simulink model "multirotor_sim"  (R2021a)
settings: Solver=ode45  StartTime=0.0  StopTime=10  RelTol=1e-9  SampleTimeConstraint=STIndependent
values from neighbouring files (symbols this model uses):
  framePeriod_s = 1/frameRate_hz    (= 0.02)    [autocode_setup.m]    (also in setup.m)
undefined symbols (not defined in the file or in its folder): Aircraft, datetime, datevec, Earth, Env, Fmu, InitCond, Telem, WGS84
libraries: simulink x8, aerolibconvert2 x5, simulink_extras x4, aerolibtransform2 x3, aerolibasang x3, aerolibgravity2 x2, sharedtransform x1, aerolibatmos2 x1, uavutilslib x1, shared6dof x1
(part 2 of 3)

== system multirotor_sim/Flight Management Unit/Control Laws/Variant Subsystem/FMU v2 ==
  System Data : Inport
  Sensor Data : Inport  Port=2
  Navigation Filter Data : Inport  Port=3
  Telemetry Data : Inport  Port=4
  Flight Code : ModelReference  ModelNameDialog=fmu_v2.slx  SimulationMode=Normal  ModelReferenceVersion=2.2
  Virtual to Non-Virtual Mapping : Subsystem
  Virtual to Non-Virtual Mapping1 : Subsystem
  Virtual to Non-Virtual Mapping2 : Subsystem
  Virtual to Non-Virtual Mapping3 : Subsystem
  Virtual to Non-Virtual Mapping4 : Subsystem
  Control Data : Outport
  wires:
  Virtual to Non-Virtual Mapping3/1(Non-Virtual) -> Flight Code/4
  Sensor Data/1 -> Virtual to Non-Virtual Mapping1/1(Virtual)
  Virtual to Non-Virtual Mapping4/1(Virtual) -> Control Data/1
  Virtual to Non-Virtual Mapping/1(Non-Virtual) -> Flight Code/1
  Flight Code/1 -> Virtual to Non-Virtual Mapping4/1(Non-Virtual)
  System Data/1 -> Virtual to Non-Virtual Mapping/1(Virtual)
  Navigation Filter Data/1 -> Virtual to Non-Virtual Mapping2/1(Virtual)
  Virtual to Non-Virtual Mapping1/1(Non-Virtual) -> Flight Code/2
  Virtual to Non-Virtual Mapping2/1(Non-Virtual) -> Flight Code/3
  Telemetry Data/1 -> Virtual to Non-Virtual Mapping3/1(Virtual)

== system multirotor_sim/Flight Management Unit/Control Laws/Variant Subsystem/FMU v2 Beta ==
  System Data : Inport
  Sensor Data : Inport  Port=2
  Navigation Filter Data : Inport  Port=3
  Telemetry Data : Inport  Port=4
  Flight Code : ModelReference  ModelNameDialog=fmu_v2_beta.slx  SimulationMode=Normal  ModelReferenceVersion=2.1
  Virtual to Non-Virtual Mapping : Subsystem
  Virtual to Non-Virtual Mapping1 : Subsystem
  Virtual to Non-Virtual Mapping2 : Subsystem
  Virtual to Non-Virtual Mapping3 : Subsystem
  Virtual to Non-Virtual Mapping4 : Subsystem
  Control Data : Outport
  wires:
  Virtual to Non-Virtual Mapping3/1(Non-Virtual) -> Flight Code/4
  Sensor Data/1 -> Virtual to Non-Virtual Mapping1/1(Virtual)
  Virtual to Non-Virtual Mapping4/1(Virtual) -> Control Data/1
  Virtual to Non-Virtual Mapping/1(Non-Virtual) -> Flight Code/1
  Flight Code/1 -> Virtual to Non-Virtual Mapping4/1(Non-Virtual)
  System Data/1 -> Virtual to Non-Virtual Mapping/1(Virtual)
  Navigation Filter Data/1 -> Virtual to Non-Virtual Mapping2/1(Virtual)
  Virtual to Non-Virtual Mapping1/1(Non-Virtual) -> Flight Code/2
  Virtual to Non-Virtual Mapping2/1(Non-Virtual) -> Flight Code/3
  Telemetry Data/1 -> Virtual to Non-Virtual Mapping3/1(Virtual)

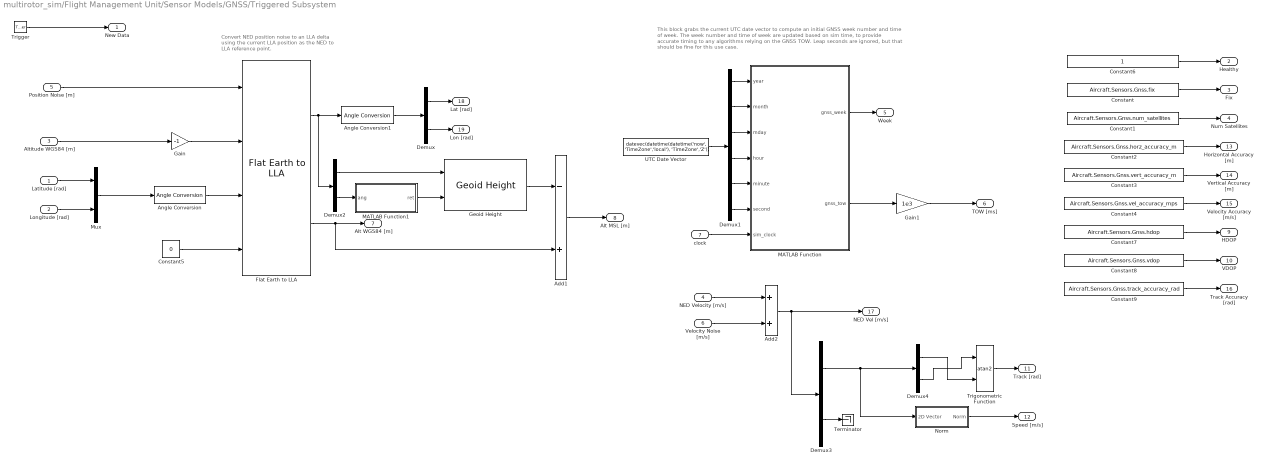
== system multirotor_sim/Flight Management Unit/Sensor Models/GNSS/Triggered Subsystem ==
  note: This block grabs the current UTC date vector to compute an initial GNSS week number
      | and time of week. The week number and time of week are updated based on sim time, to provide accurate timing to any algorithms relying on the GNSS TOW. Leap seconds are ignored, but that should be fine for this use case.
  note: Convert NED position noise to an LLA delta
      | using the current LLA position as the NED to
      | LLA reference point.
  Latitude [rad] : Inport
  "Longitude [rad] " : Inport  Port=2
  Altitude WGS84 [m] : Inport  Port=3
  NED Velocity [m/s] : Inport  Port=4  PortDimensions=3
  Position Noise [m] : Inport  Port=5  PortDimensions=3
  Velocity Noise [m/s] : Inport  Port=6  PortDimensions=3
  clock : Inport  Port=7
  Trigger : TriggerPort  VariantControl=Variant  ShowOutputPort=on
  Add1 : Sum  Inputs=-+
  Add2 : Sum
  Angle Conversion : aerolibconvert2/Angle Conversion  IU=rad  OU=deg
  Angle Conversion1 : aerolibconvert2/Angle Conversion  IU=deg  OU=rad
  Constant : Constant  Value=Aircraft.Sensors.Gnss.fix
  Constant1 : Constant  Value=Aircraft.Sensors.Gnss.num_satellites
  Constant2 : Constant  Value=Aircraft.Sensors.Gnss.horz_accuracy_m
  Constant3 : Constant  Value=Aircraft.Sensors.Gnss.vert_accuracy_m
  Constant4 : Constant  Value=Aircraft.Sensors.Gnss.vel_accuracy_mps
  Constant5 : Constant  Value=0
  Constant6 : Constant
  Constant7 : Constant  Value=Aircraft.Sensors.Gnss.hdop
  Constant8 : Constant  Value=Aircraft.Sensors.Gnss.vdop
  Constant9 : Constant  Value=Aircraft.Sensors.Gnss.track_accuracy_rad
  Demux : Demux  Outputs=2
  Demux1 : Demux  Outputs=6
  Demux2 : Demux  Outputs=2
  Demux3 : Demux  Outputs=[2 1]
  Demux4 : Demux  Outputs=2
  Flat Earth to LLA : aerolibtransform2/Flat Earth to LLA  units=Metric (MKS)  ptype=Earth (WGS84)  F=1/298.257223563  R=6378137  refPosPort=on  LL0=[0 10]  psi=0
  Gain : Gain  Gain=-1
  Gain1 : Gain  Gain=1e3
  Geoid Height : aerolibgravity2/Geoid Height  units=Metric (MKS)  gtype=EGM96  datafile='geoidegm96grid'  dtype=double  action=Warning
      settings: SourceProductBaseCode=AE
  MATLAB Function : MATLAB Function  TreatAsAtomicUnit=on
  MATLAB Function1 : MATLAB Function  TreatAsAtomicUnit=on
  Mux : Mux  Inputs=2
  Norm : Subsystem
  Terminator : Terminator
  Trigonometric Function : Trigonometry  Operator=atan2
  UTC Date Vector : Constant  Value=datevec(datetime(datetime('now', 'TimeZone','local'), 'TimeZone','Z'))  SampleTime=-1
  New Data : Outport
  Healthy : Outport  Port=2
  Fix : Outport  Port=3
  Num Satellites : Outport  Port=4
  Week : Outport  Port=5
  TOW [ms] : Outport  Port=6
  Alt WGS84 [m] : Outport  Port=7
  Alt MSL [m] : Outport  Port=8
  HDOP : Outport  Port=9
  VDOP : Outport  Port=10
  Track [rad] : Outport  Port=11
  Speed [m/s] : Outport  Port=12
  Horizontal Accuracy [m] : Outport  Port=13
  Vertical Accuracy [m] : Outport  Port=14
  Velocity Accuracy [m/s] : Outport  Port=15
  Track Accuracy [rad] : Outport  Port=16
  NED Vel [m/s] : Outport  Port=17
  Lat [rad] : Outport  Port=18
  Lon [rad] : Outport  Port=19
  wires:
  Constant/1 -> Fix/1
  Constant1/1 -> Num Satellites/1
  Constant2/1 -> Horizontal Accuracy [m]/1
  Constant3/1 -> Vertical Accuracy [m]/1
  Constant4/1 -> Velocity Accuracy [m/s]/1
  Position Noise [m]/1 -> Flat Earth to LLA/1
  Altitude WGS84 [m]/1 -> Gain/1
  Mux/1 -> Angle Conversion/1
  Angle Conversion/1 -> Flat Earth to LLA/3
  Constant5/1 -> Flat Earth to LLA/4
  "Longitude [rad] "/1 -> Mux/2
  Latitude [rad]/1 -> Mux/1
  Flat Earth to LLA/1 -> Demux2/1, Angle Conversion1/1
  Angle Conversion1/1 -> Demux/1
  Demux/2 -> Lon [rad]/1
  Demux/1 -> Lat [rad]/1
  Flat Earth to LLA/2 -> Add1/2, Alt WGS84 [m]/1
  NED Velocity [m/s]/1 -> Add2/1
  Add2/1 -> Demux3/1, NED Vel [m/s]/1
  Demux1/2 -> MATLAB Function/2(month)
  Demux1/6 -> MATLAB Function/6(second)
  UTC Date Vector/1 -> Demux1/1
  Demux1/1 -> MATLAB Function/1(year)
  Demux1/5 -> MATLAB Function/5(minute)
  Demux1/4 -> MATLAB Function/4(hour)
  Demux1/3 -> MATLAB Function/3(mday)
  MATLAB Function/2(gnss_tow) -> Gain1/1
  MATLAB Function/1(gnss_week) -> Week/1
  clock/1 -> MATLAB Function/7(sim_clock)
  Gain/1 -> Flat Earth to LLA/2
  Constant6/1 -> Healthy/1
  Trigger/1 -> New Data/1
  Gain1/1 -> TOW [ms]/1
  Demux2/1 -> Geoid Height/1
  Demux2/2 -> MATLAB Function1/1(ang)
  MATLAB Function1/1(ret) -> Geoid Height/2
  Geoid Height/1 -> Add1/1
  Add1/1 -> Alt MSL [m]/1
  Constant7/1 -> HDOP/1
  Constant8/1 -> VDOP/1
  Demux4/1 -> Trigonometric Function/2
  Demux4/2 -> Trigonometric Function/1
  Trigonometric Function/1 -> Track [rad]/1
  Velocity Noise [m/s]/1 -> Add2/2
  Constant9/1 -> Track Accuracy [rad]/1
  Demux3/1 -> Norm/1(2D Vector), Demux4/1
  Demux3/2 -> Terminator/1
  Norm/1(Norm) -> Speed [m/s]/1

== system multirotor_sim/Flight Management Unit/Sensor Models/IMU/Accelerometer ==
  Body Accel [m/s/s] : Inport  PortDimensions=3
  Gravitational Accel in Body Frame [m/s/s] : Inport  Port=2  PortDimensions=3
  Add : Sum  Inputs=+++
  Band-Limited White Noise : simulink/Sources/Band-Limited White Noise  Cov=Aircraft.Sensors.Imu.Accel.noise_mps2  Ts=0.1  seed=[23341]
  Constant : Constant  Value=Aircraft.Sensors.Imu.Accel.bias_mps2  VectorParams1D=off
  Constant1 : Constant  Value=Aircraft.Sensors.Imu.Accel.scale_factor
  Product : Product  Multiplication=Matrix(*)
  Reshape : Reshape  OutputDimensionality=Column vector (2-D)
  Reshape1 : Reshape  OutputDimensionality=Column vector (2-D)
  Reshape2 : Reshape
  Saturation : Saturate  UpperLimit=Aircraft.Sensors.Imu.Accel.upper_limit_mps2  LowerLimit=Aircraft.Sensors.Imu.Accel.lower_limit_mps2
  Subtract : Sum  Inputs=+-
  Accelerometer [m/s/s] : Outport  PortDimensions=3
  wires:
  Add/1 -> Saturation/1
  Band-Limited White Noise/1 -> Add/1
  Product/1 -> Add/3
  Constant/1 -> Add/2
  Constant1/1 -> Product/1
  Subtract/1 -> Product/2
  Reshape/1 -> Subtract/2
  Gravitational Accel in Body Frame [m/s/s]/1 -> Reshape/1
  Reshape1/1 -> Subtract/1
  Body Accel [m/s/s]/1 -> Reshape1/1
  Saturation/1 -> Reshape2/1
  Reshape2/1 -> Accelerometer [m/s/s]/1

== system multirotor_sim/Flight Management Unit/Sensor Models/IMU/Gyro ==
  Body Rotational Rate [rad/s] : Inport  PortDimensions=3
  Body Accel [m/s/s] : Inport  Port=2  PortDimensions=3
  Add1 : Sum  Inputs=++++
  Band-Limited White Noise : simulink/Sources/Band-Limited White Noise  Cov=Aircraft.Sensors.Imu.Gyro.noise_radps  Ts=0.1  seed=[23341]  VectorParams1D=off
  Constant1 : Constant  Value=Aircraft.Sensors.Imu.Gyro.bias_radps  VectorParams1D=off
  Constant2 : Constant  Value=Aircraft.Sensors.Imu.Gyro.accel_sens_radps
  Constant3 : Constant  Value=Aircraft.Sensors.Imu.Gyro.scale_factor  VectorParams1D=off
  Product : Product
  Product1 : Product  Multiplication=Matrix(*)
  Reshape : Reshape  OutputDimensionality=Column vector (2-D)
  Reshape1 : Reshape  OutputDimensionality=Column vector (2-D)
  Reshape2 : Reshape
  Saturation : Saturate  UpperLimit=Aircraft.Sensors.Imu.Gyro.upper_limit_radps  LowerLimit=Aircraft.Sensors.Imu.Gyro.lower_limit_radps
  Gyro [rad/s] : Outport  PortDimensions=3
  wires:
  Constant3/1 -> Product1/1
  Constant2/1 -> Product/1
  Add1/1 -> Saturation/1
  Constant1/1 -> Add1/3
  Product1/1 -> Add1/4
  Band-Limited White Noise/1 -> Add1/2
  Body Rotational Rate [rad/s]/1 -> Reshape/1
  Reshape/1 -> Product1/2
  Body Accel [m/s/s]/1 -> Product/2
  Product/1 -> Reshape1/1
  Reshape1/1 -> Add1/1
  Reshape2/1 -> Gyro [rad/s]/1
  Saturation/1 -> Reshape2/1

== system multirotor_sim/Flight Management Unit/Sensor Models/IMU/Magnetometer ==
  Body Magnetic Field [uT] : Inport  PortDimensions=3
  Add2 : Sum  Inputs=+++
  Band-Limited White Noise : simulink/Sources/Band-Limited White Noise  Cov=Aircraft.Sensors.Imu.Mag.noise_ut  Ts=0.1  seed=[23341]
  Constant1 : Constant  Value=Aircraft.Sensors.Imu.Mag.scale_factor  VectorParams1D=off
  Constant2 : Constant  Value=Aircraft.Sensors.Imu.Mag.bias_ut
  Product : Product  Multiplication=Matrix(*)
  Reshape : Reshape  OutputDimensionality=Column vector (2-D)
  Reshape1 : Reshape
  Saturation : Saturate  UpperLimit=Aircraft.Sensors.Imu.Mag.upper_limit_ut  LowerLimit=Aircraft.Sensors.Imu.Mag.lower_limit_ut
  Magnetometer [uT] : Outport  PortDimensions=3
  wires:
  Body Magnetic Field [uT]/1 -> Reshape/1
  Band-Limited White Noise/1 -> Add2/1
  Add2/1 -> Saturation/1
  Constant2/1 -> Add2/2
  Constant1/1 -> Product/1
  Reshape/1 -> Product/2
  Saturation/1 -> Reshape1/1
  Reshape1/1 -> Magnetometer [uT]/1
  Product/1 -> Add2/3

== system multirotor_sim/Vehicle/Forces and Moments/Propulsive/Mz calculation1 ==
  Motor_torque : Inport
  Constant : Constant  Value=Aircraft.Motor.dir
  MatrixMultiply : Product  Multiplication=Matrix(*)
  Mz_from_motor_torque : Outport
  wires:
  Motor_torque/1 -> MatrixMultiply/1
  Constant/1 -> MatrixMultiply/2
  MatrixMultiply/1 -> Mz_from_motor_torque/1

== system multirotor_sim/Flight Management Unit/Control Laws/Variant Subsystem/FMU v1/Virtual to Non-Virtual Mapping ==
  Virtual : Inport
  Bus Creator : BusCreator  Inputs=8  OutDataTypeStr=Bus: SysData  NonVirtualBus=on
  Bus Selector : BusSelector  OutputSignals=Frame Time [us],Frame Time [s],Input Voltage,Regulated Voltage,PWM Voltage,SBUS Voltage,System Time [us],System Time [s]
  Data Type Conversion : DataTypeConversion  OutDataTypeStr=int32
  Data Type Conversion{1..4,6} (5 alike) : DataTypeConversion  OutDataTypeStr=single
  Data Type Conversion5 : DataTypeConversion  OutDataTypeStr=int64
  Data Type Conversion7 : DataTypeConversion  OutDataTypeStr=double
  Non-Virtual : Outport  OutDataTypeStr=Bus: SysData
  wires:
  Data Type Conversion7/1 -> Bus Creator/8  "sys_time_s"
  Bus Selector/8 -> Data Type Conversion7/1  "<System Time [s]>"
  Data Type Conversion6/1 -> Bus Creator/2  "frame_time_s"
  Bus Selector/2 -> Data Type Conversion6/1  "<Frame Time [s]>"
  Data Type Conversion5/1 -> Bus Creator/7  "sys_time_us"
  Bus Selector/7 -> Data Type Conversion5/1  "<System Time [us]>"
  Data Type Conversion4/1 -> Bus Creator/6  "sbus_volt"
  Data Type Conversion3/1 -> Bus Creator/5  "pwm_volt"
  Data Type Conversion2/1 -> Bus Creator/4  "reg_volt"
  Bus Selector/6 -> Data Type Conversion4/1  "<SBUS Voltage>"
  Bus Selector/5 -> Data Type Conversion3/1  "<PWM Voltage>"
  Bus Selector/4 -> Data Type Conversion2/1  "<Regulated Voltage>"
  Data Type Conversion1/1 -> Bus Creator/3  "input_volt"
  Bus Selector/3 -> Data Type Conversion1/1  "<Input Voltage>"
  Data Type Conversion/1 -> Bus Creator/1  "frame_time_us"
  Bus Selector/1 -> Data Type Conversion/1  "<Frame Time [us]>"
  Virtual/1 -> Bus Selector/1
  Bus Creator/1 -> Non-Virtual/1

== system multirotor_sim/Flight Management Unit/Control Laws/Variant Subsystem/FMU v1/Virtual to Non-Virtual Mapping1 ==
  Virtual : Inport
  Bus Creator : BusCreator  Inputs=7  OutDataTypeStr=Bus: SensorData  NonVirtualBus=on
  Bus Selector : BusSelector  OutputSignals=Pitot Static Installed,Inceptor,IMU,GNSS,Static Pressure,Differential Pressure,Analog
  Data Type Conversion : DataTypeConversion  OutDataTypeStr=boolean
  Virtual to Non-Virtual Mapping1 : Subsystem
  Virtual to Non-Virtual Mapping2 : Subsystem
  Virtual to Non-Virtual Mapping3 : Subsystem
  Virtual to Non-Virtual Mapping4 : Subsystem
  Virtual to Non-Virtual Mapping5 : Subsystem
  Virtual to Non-Virtual Mapping6 : Subsystem
  Non-Virtual : Outport  OutDataTypeStr=Bus: SensorData
  wires:
  Virtual to Non-Virtual Mapping6/1(Non-Virtual) -> Bus Creator/7  "analog"
  Bus Selector/7 -> Virtual to Non-Virtual Mapping6/1(Virtual)  "<Analog>"
  Bus Selector/6 -> Virtual to Non-Virtual Mapping5/1(Virtual)  "<Differential Pressure>"
  Virtual to Non-Virtual Mapping5/1(Non-Virtual) -> Bus Creator/6  "diff_pres"
  Bus Selector/5 -> Virtual to Non-Virtual Mapping4/1(Virtual)  "<Static Pressure>"
  Virtual to Non-Virtual Mapping4/1(Non-Virtual) -> Bus Creator/5  "static_pres"
  Bus Selector/4 -> Virtual to Non-Virtual Mapping3/1(Virtual)  "<GNSS>"
  Virtual to Non-Virtual Mapping3/1(Non-Virtual) -> Bus Creator/4  "gnss"
  Bus Selector/3 -> Virtual to Non-Virtual Mapping2/1(Virtual)  "<IMU>"
  Virtual to Non-Virtual Mapping2/1(Non-Virtual) -> Bus Creator/3  "imu"
  Virtual to Non-Virtual Mapping1/1(Non-Virtual) -> Bus Creator/2  "inceptor"
  Bus Selector/2 -> Virtual to Non-Virtual Mapping1/1(Virtual)  "<Inceptor>"
  Data Type Conversion/1 -> Bus Creator/1  "pitot_static_installed"
  Bus Selector/1 -> Data Type Conversion/1  "<Pitot Static Installed>"
  Bus Creator/1 -> Non-Virtual/1
  Virtual/1 -> Bus Selector/1

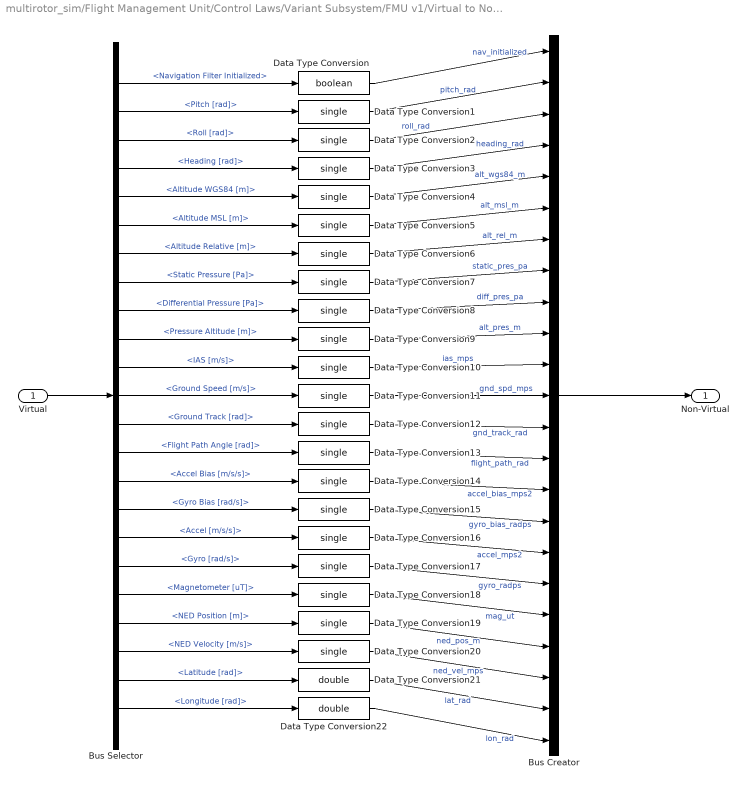
== system multirotor_sim/Flight Management Unit/Control Laws/Variant Subsystem/FMU v1/Virtual to Non-Virtual Mapping2 ==
  Virtual : Inport
  Bus Creator : BusCreator  Inputs=23  OutDataTypeStr=Bus: NavData  NonVirtualBus=on
  Bus Selector : BusSelector  OutputSignals=Navigation Filter Initialized,Pitch [rad],Roll [rad],Heading [rad],Altitude WGS84 [m],Altitude MSL [m],Altitude Relative [m],Static Pressure [Pa],Differential Pressure [Pa],Pressure Altitude [m],IAS [m/s],Ground Speed [m/s],Ground Track [rad],Flight Path Angle [rad],Accel Bias [m/s/s],Gyro Bias [rad/s],Accel [m/s/s],Gyro [rad/s],Magnetometer [uT],NED Position [m],NED Velocity [m/s],Latitude [rad],Longitude [rad]
  Data Type Conversion : DataTypeConversion  OutDataTypeStr=boolean
  Data Type Conversion{1..20} (20 alike) : DataTypeConversion  OutDataTypeStr=single
  Data Type Conversion21 : DataTypeConversion  OutDataTypeStr=double
  Data Type Conversion22 : DataTypeConversion  OutDataTypeStr=double
  Non-Virtual : Outport  OutDataTypeStr=Bus: NavData
  wires:
  Data Type Conversion17/1 -> Bus Creator/18  "gyro_radps"
  Data Type Conversion22/1 -> Bus Creator/23  "lon_rad"
  Data Type Conversion21/1 -> Bus Creator/22  "lat_rad"
  Data Type Conversion20/1 -> Bus Creator/21  "ned_vel_mps"
  Data Type Conversion19/1 -> Bus Creator/20  "ned_pos_m"
  Data Type Conversion18/1 -> Bus Creator/19  "mag_ut"
  Data Type Conversion16/1 -> Bus Creator/17  "accel_mps2"
  Data Type Conversion15/1 -> Bus Creator/16  "gyro_bias_radps"
  Data Type Conversion14/1 -> Bus Creator/15  "accel_bias_mps2"
  Data Type Conversion13/1 -> Bus Creator/14  "flight_path_rad"
  Data Type Conversion12/1 -> Bus Creator/13  "gnd_track_rad"
  Data Type Conversion11/1 -> Bus Creator/12  "gnd_spd_mps"
  Data Type Conversion10/1 -> Bus Creator/11  "ias_mps"
  Data Type Conversion9/1 -> Bus Creator/10  "alt_pres_m"
  Data Type Conversion8/1 -> Bus Creator/9  "diff_pres_pa"
  Data Type Conversion7/1 -> Bus Creator/8  "static_pres_pa"
  Data Type Conversion6/1 -> Bus Creator/7  "alt_rel_m"
  Data Type Conversion5/1 -> Bus Creator/6  "alt_msl_m"
  Data Type Conversion4/1 -> Bus Creator/5  "alt_wgs84_m"
  Data Type Conversion3/1 -> Bus Creator/4  "heading_rad"
  Data Type Conversion2/1 -> Bus Creator/3  "roll_rad"
  Data Type Conversion1/1 -> Bus Creator/2  "pitch_rad"
  Data Type Conversion/1 -> Bus Creator/1  "nav_initialized"
  Bus Selector/23 -> Data Type Conversion22/1  "<Longitude [rad]>"
  Bus Selector/22 -> Data Type Conversion21/1  "<Latitude [rad]>"
  Bus Selector/21 -> Data Type Conversion20/1  "<NED Velocity [m/s]>"
  Bus Selector/20 -> Data Type Conversion19/1  "<NED Position [m]>"
  Bus Selector/19 -> Data Type Conversion18/1  "<Magnetometer [uT]>"
  Bus Selector/18 -> Data Type Conversion17/1  "<Gyro [rad/s]>"
  Bus Selector/17 -> Data Type Conversion16/1  "<Accel [m/s/s]>"
  Bus Selector/16 -> Data Type Conversion15/1  "<Gyro Bias [rad/s]>"
  Bus Selector/15 -> Data Type Conversion14/1  "<Accel Bias [m/s/s]>"
  Bus Selector/14 -> Data Type Conversion13/1  "<Flight Path Angle [rad]>"
  Bus Selector/13 -> Data Type Conversion12/1  "<Ground Track [rad]>"
  Bus Selector/12 -> Data Type Conversion11/1  "<Ground Speed [m/s]>"
  Bus Selector/11 -> Data Type Conversion10/1  "<IAS [m/s]>"
  Bus Selector/10 -> Data Type Conversion9/1  "<Pressure Altitude [m]>"
  Bus Selector/9 -> Data Type Conversion8/1  "<Differential Pressure [Pa]>"
  Bus Selector/8 -> Data Type Conversion7/1  "<Static Pressure [Pa]>"
  Bus Selector/7 -> Data Type Conversion6/1  "<Altitude Relative [m]>"
  Bus Selector/6 -> Data Type Conversion5/1  "<Altitude MSL [m]>"
  Bus Selector/5 -> Data Type Conversion4/1  "<Altitude WGS84 [m]>"
  Bus Selector/4 -> Data Type Conversion3/1  "<Heading [rad]>"
  Bus Selector/3 -> Data Type Conversion2/1  "<Roll [rad]>"
  Bus Selector/2 -> Data Type Conversion1/1  "<Pitch [rad]>"
  Bus Selector/1 -> Data Type Conversion/1  "<Navigation Filter Initialized>"
  Bus Creator/1 -> Non-Virtual/1
  Virtual/1 -> Bus Selector/1

== system multirotor_sim/Flight Management Unit/Control Laws/Variant Subsystem/FMU v1/Virtual to Non-Virtual Mapping3 ==
  Virtual : Inport
  Bus Creator : BusCreator  Inputs=11  OutDataTypeStr=Bus: TelemData  NonVirtualBus=on
  Bus Selector : BusSelector  OutputSignals=Waypoints Updated,Fence Updated,Rally Points Updated,Current Waypoint Index,Number of Waypoints,Number of Fence Points,Number of Rally Points,Parameters,Flight Plan,Fence,Rally
  Data Type Conversion : DataTypeConversion  OutDataTypeStr=boolean
  Data Type Conversion1 : DataTypeConversion  OutDataTypeStr=boolean
  Data Type Conversion2 : DataTypeConversion  OutDataTypeStr=boolean
  Data Type Conversion{3..6} (4 alike) : DataTypeConversion  OutDataTypeStr=int16
  Data Type Conversion7 : DataTypeConversion  OutDataTypeStr=single
  Signal Conversion : SignalConversion  ConversionOutput=Nonvirtual bus  OverrideOpt=off
  Signal Conversion1 : SignalConversion  ConversionOutput=Nonvirtual bus  OverrideOpt=off
  Signal Conversion2 : SignalConversion  ConversionOutput=Nonvirtual bus  OverrideOpt=off
  Non-Virtual : Outport  OutDataTypeStr=Bus: TelemData
  wires:
  Signal Conversion2/1 -> Bus Creator/11  "rally"
  Signal Conversion1/1 -> Bus Creator/10  "fence"
  Signal Conversion/1 -> Bus Creator/9  "flight_plan"
  Bus Selector/11 -> Signal Conversion2/1  "<Rally>"
  Bus Selector/10 -> Signal Conversion1/1  "<Fence>"
  Bus Selector/9 -> Signal Conversion/1  "<Flight Plan>"
  Data Type Conversion7/1 -> Bus Creator/8  "param"
  Data Type Conversion6/1 -> Bus Creator/7  "num_rally_points"
  Data Type Conversion5/1 -> Bus Creator/6  "num_fence_items"
  Data Type Conversion4/1 -> Bus Creator/5  "num_waypoints"
  Data Type Conversion3/1 -> Bus Creator/4  "current_waypoint"
  Data Type Conversion2/1 -> Bus Creator/3  "rally_points_updated"
  Data Type Conversion1/1 -> Bus Creator/2  "fence_updated"
  Data Type Conversion/1 -> Bus Creator/1  "waypoints_updated"
  Bus Selector/8 -> Data Type Conversion7/1  "<Parameters>"
  Bus Selector/7 -> Data Type Conversion6/1  "<Number of Rally Points>"
  Bus Selector/6 -> Data Type Conversion5/1  "<Number of Fence Points>"
  Bus Selector/5 -> Data Type Conversion4/1  "<Number of Waypoints>"
  Bus Selector/4 -> Data Type Conversion3/1  "<Current Waypoint Index>"
  Bus Selector/3 -> Data Type Conversion2/1  "<Rally Points Updated>"
  Bus Selector/2 -> Data Type Conversion1/1  "<Fence Updated>"
  Bus Selector/1 -> Data Type Conversion/1  "<Waypoints Updated>"
  Bus Creator/1 -> Non-Virtual/1
  Virtual/1 -> Bus Selector/1

== system multirotor_sim/Flight Management Unit/Control Laws/Variant Subsystem/FMU v1/Virtual to Non-Virtual Mapping4 ==
  Non-Virtual : Inport  OutDataTypeStr=Bus: ControlData
  Bus Creator : BusCreator  Inputs=5
  Bus Selector : BusSelector  OutputSignals=waypoint_reached,mode,sbus,pwm,aux
  Data Type Conversion{1..4,22} (5 alike) : DataTypeConversion  OutDataTypeStr=double
  Virtual : Outport
  wires:
  Data Type Conversion4/1 -> Bus Creator/5  "AUX"
  Data Type Conversion3/1 -> Bus Creator/4  "PWM"
  Bus Selector/5 -> Data Type Conversion4/1  "<aux>"
  Bus Selector/4 -> Data Type Conversion3/1  "<pwm>"
  Data Type Conversion2/1 -> Bus Creator/3  "SBUS"
  Bus Selector/3 -> Data Type Conversion2/1  "<sbus>"
  Data Type Conversion1/1 -> Bus Creator/2  "Mode"
  Bus Selector/2 -> Data Type Conversion1/1  "<mode>"
  Data Type Conversion22/1 -> Bus Creator/1  "Waypoint Reached"
  Bus Selector/1 -> Data Type Conversion22/1  "<waypoint_reached>"
  Bus Creator/1 -> Virtual/1
  Non-Virtual/1 -> Bus Selector/1

== system multirotor_sim/Flight Management Unit/Control Laws/Variant Subsystem/FMU v2/Virtual to Non-Virtual Mapping ==
  Virtual : Inport
  Bus Creator : BusCreator  Inputs=4  OutDataTypeStr=Bus: SysData  NonVirtualBus=on
  Bus Selector : BusSelector  OutputSignals=Frame Time [us],Frame Time [s],System Time [us],System Time [s]
  Data Type Conversion : DataTypeConversion  OutDataTypeStr=int32
  Data Type Conversion5 : DataTypeConversion  OutDataTypeStr=int64
  Data Type Conversion6 : DataTypeConversion  OutDataTypeStr=single
  Data Type Conversion7 : DataTypeConversion  OutDataTypeStr=double
  Non-Virtual : Outport  OutDataTypeStr=Bus: SysData
  wires:
  Bus Creator/1 -> Non-Virtual/1
  Virtual/1 -> Bus Selector/1
  Bus Selector/1 -> Data Type Conversion/1  "<Frame Time [us]>"
  Data Type Conversion/1 -> Bus Creator/1  "frame_time_us"
  Bus Selector/3 -> Data Type Conversion5/1  "<System Time [us]>"
  Data Type Conversion5/1 -> Bus Creator/3  "sys_time_us"
  Bus Selector/2 -> Data Type Conversion6/1  "<Frame Time [s]>"
  Data Type Conversion6/1 -> Bus Creator/2  "frame_time_s"
  Bus Selector/4 -> Data Type Conversion7/1  "<System Time [s]>"
  Data Type Conversion7/1 -> Bus Creator/4  "sys_time_s"

== system multirotor_sim/Flight Management Unit/Control Laws/Variant Subsystem/FMU v2/Virtual to Non-Virtual Mapping1 ==
  Virtual : Inport
  Bus Creator : BusCreator  Inputs=8  OutDataTypeStr=Bus: SensorData  NonVirtualBus=on
  Bus Selector : BusSelector  OutputSignals=Pitot Static Installed,Inceptor,IMU,GNSS,Static Pressure,Differential Pressure,Analog,Battery
  Data Type Conversion : DataTypeConversion  OutDataTypeStr=boolean
  Virtual to Non-Virtual Mapping1 : Subsystem
  Virtual to Non-Virtual Mapping2 : Subsystem
  Virtual to Non-Virtual Mapping3 : Subsystem
  Virtual to Non-Virtual Mapping4 : Subsystem
  Virtual to Non-Virtual Mapping5 : Subsystem
  Virtual to Non-Virtual Mapping6 : Subsystem
  Virtual to Non-Virtual Mapping7 : Subsystem
  Non-Virtual : Outport  OutDataTypeStr=Bus: SensorData
  wires:
  Virtual/1 -> Bus Selector/1
  Bus Creator/1 -> Non-Virtual/1
  Bus Selector/1 -> Data Type Conversion/1  "<Pitot Static Installed>"
  Data Type Conversion/1 -> Bus Creator/1  "pitot_static_installed"
  Bus Selector/2 -> Virtual to Non-Virtual Mapping1/1(Virtual)  "<Inceptor>"
  Virtual to Non-Virtual Mapping1/1(Non-Virtual) -> Bus Creator/2  "inceptor"
  Virtual to Non-Virtual Mapping2/1(Non-Virtual) -> Bus Creator/3  "imu"
  Bus Selector/3 -> Virtual to Non-Virtual Mapping2/1(Virtual)  "<IMU>"
  Virtual to Non-Virtual Mapping3/1(Non-Virtual) -> Bus Creator/4  "gnss"
  Bus Selector/4 -> Virtual to Non-Virtual Mapping3/1(Virtual)  "<GNSS>"
  Virtual to Non-Virtual Mapping4/1(Non-Virtual) -> Bus Creator/5  "static_pres"
  Bus Selector/5 -> Virtual to Non-Virtual Mapping4/1(Virtual)  "<Static Pressure>"
  Virtual to Non-Virtual Mapping5/1(Non-Virtual) -> Bus Creator/6  "diff_pres"
  Bus Selector/6 -> Virtual to Non-Virtual Mapping5/1(Virtual)  "<Differential Pressure>"
  Bus Selector/7 -> Virtual to Non-Virtual Mapping6/1(Virtual)  "<Analog>"
  Virtual to Non-Virtual Mapping6/1(Non-Virtual) -> Bus Creator/7  "analog"
  Virtual to Non-Virtual Mapping7/1(Non-Virtual) -> Bus Creator/8  "battery"
  Bus Selector/8 -> Virtual to Non-Virtual Mapping7/1(Virtual)  "<Battery>"

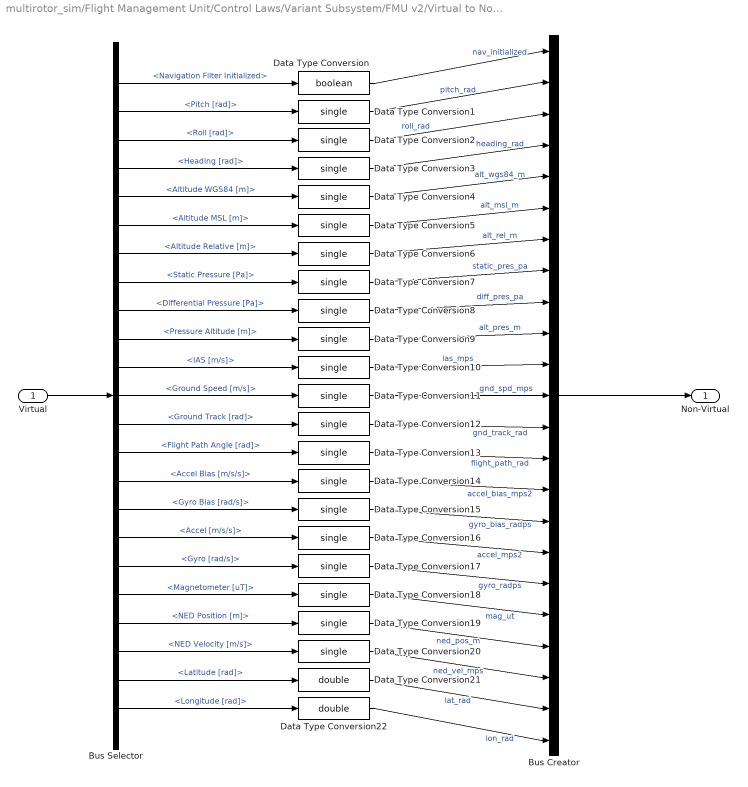
== system multirotor_sim/Flight Management Unit/Control Laws/Variant Subsystem/FMU v2/Virtual to Non-Virtual Mapping2 ==
  Virtual : Inport
  Bus Creator : BusCreator  Inputs=23  OutDataTypeStr=Bus: NavData  NonVirtualBus=on
  Bus Selector : BusSelector  OutputSignals=Navigation Filter Initialized,Pitch [rad],Roll [rad],Heading [rad],Altitude WGS84 [m],Altitude MSL [m],Altitude Relative [m],Static Pressure [Pa],Differential Pressure [Pa],Pressure Altitude [m],IAS [m/s],Ground Speed [m/s],Ground Track [rad],Flight Path Angle [rad],Accel Bias [m/s/s],Gyro Bias [rad/s],Accel [m/s/s],Gyro [rad/s],Magnetometer [uT],NED Position [m],NED Velocity [m/s],Latitude [rad],Longitude [rad]
  Data Type Conversion : DataTypeConversion  OutDataTypeStr=boolean
  Data Type Conversion{1..20} (20 alike) : DataTypeConversion  OutDataTypeStr=single
  Data Type Conversion21 : DataTypeConversion  OutDataTypeStr=double
  Data Type Conversion22 : DataTypeConversion  OutDataTypeStr=double
  Non-Virtual : Outport  OutDataTypeStr=Bus: NavData
  wires:
  Virtual/1 -> Bus Selector/1
  Bus Creator/1 -> Non-Virtual/1
  Bus Selector/1 -> Data Type Conversion/1  "<Navigation Filter Initialized>"
  Bus Selector/2 -> Data Type Conversion1/1  "<Pitch [rad]>"
  Bus Selector/3 -> Data Type Conversion2/1  "<Roll [rad]>"
  Bus Selector/4 -> Data Type Conversion3/1  "<Heading [rad]>"
  Bus Selector/5 -> Data Type Conversion4/1  "<Altitude WGS84 [m]>"
  Bus Selector/6 -> Data Type Conversion5/1  "<Altitude MSL [m]>"
  Bus Selector/7 -> Data Type Conversion6/1  "<Altitude Relative [m]>"
  Bus Selector/8 -> Data Type Conversion7/1  "<Static Pressure [Pa]>"
  Bus Selector/9 -> Data Type Conversion8/1  "<Differential Pressure [Pa]>"
  Bus Selector/10 -> Data Type Conversion9/1  "<Pressure Altitude [m]>"
  Bus Selector/11 -> Data Type Conversion10/1  "<IAS [m/s]>"
  Bus Selector/12 -> Data Type Conversion11/1  "<Ground Speed [m/s]>"
  Bus Selector/13 -> Data Type Conversion12/1  "<Ground Track [rad]>"
  Bus Selector/14 -> Data Type Conversion13/1  "<Flight Path Angle [rad]>"
  Bus Selector/15 -> Data Type Conversion14/1  "<Accel Bias [m/s/s]>"
  Bus Selector/16 -> Data Type Conversion15/1  "<Gyro Bias [rad/s]>"
  Bus Selector/17 -> Data Type Conversion16/1  "<Accel [m/s/s]>"
  Bus Selector/18 -> Data Type Conversion17/1  "<Gyro [rad/s]>"
  Bus Selector/19 -> Data Type Conversion18/1  "<Magnetometer [uT]>"
  Bus Selector/20 -> Data Type Conversion19/1  "<NED Position [m]>"
  Bus Selector/21 -> Data Type Conversion20/1  "<NED Velocity [m/s]>"
  Bus Selector/22 -> Data Type Conversion21/1  "<Latitude [rad]>"
  Bus Selector/23 -> Data Type Conversion22/1  "<Longitude [rad]>"
  Data Type Conversion/1 -> Bus Creator/1  "nav_initialized"
  Data Type Conversion1/1 -> Bus Creator/2  "pitch_rad"
  Data Type Conversion2/1 -> Bus Creator/3  "roll_rad"
  Data Type Conversion3/1 -> Bus Creator/4  "heading_rad"
  Data Type Conversion4/1 -> Bus Creator/5  "alt_wgs84_m"
  Data Type Conversion5/1 -> Bus Creator/6  "alt_msl_m"
  Data Type Conversion6/1 -> Bus Creator/7  "alt_rel_m"
  Data Type Conversion7/1 -> Bus Creator/8  "static_pres_pa"
  Data Type Conversion8/1 -> Bus Creator/9  "diff_pres_pa"
  Data Type Conversion9/1 -> Bus Creator/10  "alt_pres_m"
  Data Type Conversion10/1 -> Bus Creator/11  "ias_mps"
  Data Type Conversion11/1 -> Bus Creator/12  "gnd_spd_mps"
  Data Type Conversion12/1 -> Bus Creator/13  "gnd_track_rad"
  Data Type Conversion13/1 -> Bus Creator/14  "flight_path_rad"
  Data Type Conversion14/1 -> Bus Creator/15  "accel_bias_mps2"
  Data Type Conversion15/1 -> Bus Creator/16  "gyro_bias_radps"
  Data Type Conversion16/1 -> Bus Creator/17  "accel_mps2"
  Data Type Conversion18/1 -> Bus Creator/19  "mag_ut"
  Data Type Conversion19/1 -> Bus Creator/20  "ned_pos_m"
  Data Type Conversion20/1 -> Bus Creator/21  "ned_vel_mps"
  Data Type Conversion21/1 -> Bus Creator/22  "lat_rad"
  Data Type Conversion22/1 -> Bus Creator/23  "lon_rad"
  Data Type Conversion17/1 -> Bus Creator/18  "gyro_radps"

== system multirotor_sim/Flight Management Unit/Control Laws/Variant Subsystem/FMU v2/Virtual to Non-Virtual Mapping3 ==
  Virtual : Inport
  Bus Creator : BusCreator  Inputs=11  OutDataTypeStr=Bus: TelemData  NonVirtualBus=on
  Bus Selector : BusSelector  OutputSignals=Waypoints Updated,Fence Updated,Rally Points Updated,Current Waypoint Index,Number of Waypoints,Number of Fence Points,Number of Rally Points,Parameters,Flight Plan,Fence,Rally
  Data Type Conversion : DataTypeConversion  OutDataTypeStr=boolean
  Data Type Conversion1 : DataTypeConversion  OutDataTypeStr=boolean
  Data Type Conversion2 : DataTypeConversion  OutDataTypeStr=boolean
  Data Type Conversion{3..6} (4 alike) : DataTypeConversion  OutDataTypeStr=int16
  Data Type Conversion7 : DataTypeConversion  OutDataTypeStr=single
  Signal Conversion : SignalConversion  ConversionOutput=Nonvirtual bus  OverrideOpt=off
  Signal Conversion1 : SignalConversion  ConversionOutput=Nonvirtual bus  OverrideOpt=off
  Signal Conversion2 : SignalConversion  ConversionOutput=Nonvirtual bus  OverrideOpt=off
  Non-Virtual : Outport  OutDataTypeStr=Bus: TelemData
  wires:
  Virtual/1 -> Bus Selector/1
  Bus Creator/1 -> Non-Virtual/1
  Bus Selector/1 -> Data Type Conversion/1  "<Waypoints Updated>"
  Bus Selector/2 -> Data Type Conversion1/1  "<Fence Updated>"
  Bus Selector/3 -> Data Type Conversion2/1  "<Rally Points Updated>"
  Bus Selector/4 -> Data Type Conversion3/1  "<Current Waypoint Index>"
  Bus Selector/5 -> Data Type Conversion4/1  "<Number of Waypoints>"
  Bus Selector/6 -> Data Type Conversion5/1  "<Number of Fence Points>"
  Bus Selector/7 -> Data Type Conversion6/1  "<Number of Rally Points>"
  Bus Selector/8 -> Data Type Conversion7/1  "<Parameters>"
  Data Type Conversion/1 -> Bus Creator/1  "waypoints_updated"
  Data Type Conversion1/1 -> Bus Creator/2  "fence_updated"
  Data Type Conversion2/1 -> Bus Creator/3  "rally_points_updated"
  Data Type Conversion3/1 -> Bus Creator/4  "current_waypoint"
  Data Type Conversion4/1 -> Bus Creator/5  "num_waypoints"
  Data Type Conversion5/1 -> Bus Creator/6  "num_fence_items"
  Data Type Conversion6/1 -> Bus Creator/7  "num_rally_points"
  Data Type Conversion7/1 -> Bus Creator/8  "param"
  Bus Selector/9 -> Signal Conversion/1  "<Flight Plan>"
  Bus Selector/10 -> Signal Conversion1/1  "<Fence>"
  Bus Selector/11 -> Signal Conversion2/1  "<Rally>"
  Signal Conversion/1 -> Bus Creator/9  "flight_plan"
  Signal Conversion1/1 -> Bus Creator/10  "fence"
  Signal Conversion2/1 -> Bus Creator/11  "rally"

== system multirotor_sim/Flight Management Unit/Control Laws/Variant Subsystem/FMU v2/Virtual to Non-Virtual Mapping4 ==
  Non-Virtual : Inport  OutDataTypeStr=Bus: ControlData
  Bus Creator : BusCreator  Inputs=5
  Bus Selector : BusSelector  OutputSignals=waypoint_reached,mode,sbus,pwm,aux
  Data Type Conversion{1..4,22} (5 alike) : DataTypeConversion  OutDataTypeStr=double
  Virtual : Outport
  wires:
  Non-Virtual/1 -> Bus Selector/1
  Bus Creator/1 -> Virtual/1
  Bus Selector/1 -> Data Type Conversion22/1  "<waypoint_reached>"
  Data Type Conversion22/1 -> Bus Creator/1  "Waypoint Reached"
  Bus Selector/2 -> Data Type Conversion1/1  "<mode>"
  Data Type Conversion1/1 -> Bus Creator/2  "Mode"
  Bus Selector/3 -> Data Type Conversion2/1  "<sbus>"
  Data Type Conversion2/1 -> Bus Creator/3  "SBUS"
  Bus Selector/4 -> Data Type Conversion3/1  "<pwm>"
  Bus Selector/5 -> Data Type Conversion4/1  "<aux>"
  Data Type Conversion3/1 -> Bus Creator/4  "PWM"
  Data Type Conversion4/1 -> Bus Creator/5  "AUX"

== system multirotor_sim/Flight Management Unit/Control Laws/Variant Subsystem/FMU v2 Beta/Virtual to Non-Virtual Mapping ==
  Virtual : Inport
  Bus Creator : BusCreator  Inputs=4  OutDataTypeStr=Bus: SysData  NonVirtualBus=on
  Bus Selector : BusSelector  OutputSignals=Frame Time [us],Frame Time [s],System Time [us],System Time [s]
  Data Type Conversion : DataTypeConversion  OutDataTypeStr=int32
  Data Type Conversion5 : DataTypeConversion  OutDataTypeStr=int64
  Data Type Conversion6 : DataTypeConversion  OutDataTypeStr=single
  Data Type Conversion7 : DataTypeConversion  OutDataTypeStr=double
  Non-Virtual : Outport  OutDataTypeStr=Bus: SysData
  wires:
  Bus Creator/1 -> Non-Virtual/1
  Virtual/1 -> Bus Selector/1
  Bus Selector/1 -> Data Type Conversion/1  "<Frame Time [us]>"
  Data Type Conversion/1 -> Bus Creator/1  "frame_time_us"
  Bus Selector/3 -> Data Type Conversion5/1  "<System Time [us]>"
  Data Type Conversion5/1 -> Bus Creator/3  "sys_time_us"
  Bus Selector/2 -> Data Type Conversion6/1  "<Frame Time [s]>"
  Data Type Conversion6/1 -> Bus Creator/2  "frame_time_s"
  Bus Selector/4 -> Data Type Conversion7/1  "<System Time [s]>"
  Data Type Conversion7/1 -> Bus Creator/4  "sys_time_s"

== system multirotor_sim/Flight Management Unit/Control Laws/Variant Subsystem/FMU v2 Beta/Virtual to Non-Virtual Mapping1 ==
  Virtual : Inport
  Bus Creator : BusCreator  Inputs=7  OutDataTypeStr=Bus: SensorData  NonVirtualBus=on
  Bus Selector : BusSelector  OutputSignals=Pitot Static Installed,Inceptor,IMU,GNSS,Static Pressure,Differential Pressure,Analog
  Data Type Conversion : DataTypeConversion  OutDataTypeStr=boolean
  Virtual to Non-Virtual Mapping1 : Subsystem
  Virtual to Non-Virtual Mapping2 : Subsystem
  Virtual to Non-Virtual Mapping3 : Subsystem
  Virtual to Non-Virtual Mapping4 : Subsystem
  Virtual to Non-Virtual Mapping5 : Subsystem
  Virtual to Non-Virtual Mapping6 : Subsystem
  Non-Virtual : Outport  OutDataTypeStr=Bus: SensorData
  wires:
  Virtual/1 -> Bus Selector/1
  Bus Creator/1 -> Non-Virtual/1
  Bus Selector/1 -> Data Type Conversion/1  "<Pitot Static Installed>"
  Data Type Conversion/1 -> Bus Creator/1  "pitot_static_installed"
  Bus Selector/2 -> Virtual to Non-Virtual Mapping1/1(Virtual)  "<Inceptor>"
  Virtual to Non-Virtual Mapping1/1(Non-Virtual) -> Bus Creator/2  "inceptor"
  Virtual to Non-Virtual Mapping2/1(Non-Virtual) -> Bus Creator/3  "imu"
  Bus Selector/3 -> Virtual to Non-Virtual Mapping2/1(Virtual)  "<IMU>"
  Virtual to Non-Virtual Mapping3/1(Non-Virtual) -> Bus Creator/4  "gnss"
  Bus Selector/4 -> Virtual to Non-Virtual Mapping3/1(Virtual)  "<GNSS>"
  Virtual to Non-Virtual Mapping4/1(Non-Virtual) -> Bus Creator/5  "static_pres"
  Bus Selector/5 -> Virtual to Non-Virtual Mapping4/1(Virtual)  "<Static Pressure>"
  Virtual to Non-Virtual Mapping5/1(Non-Virtual) -> Bus Creator/6  "diff_pres"
  Bus Selector/6 -> Virtual to Non-Virtual Mapping5/1(Virtual)  "<Differential Pressure>"
  Bus Selector/7 -> Virtual to Non-Virtual Mapping6/1(Virtual)  "<Analog>"
  Virtual to Non-Virtual Mapping6/1(Non-Virtual) -> Bus Creator/7  "analog"

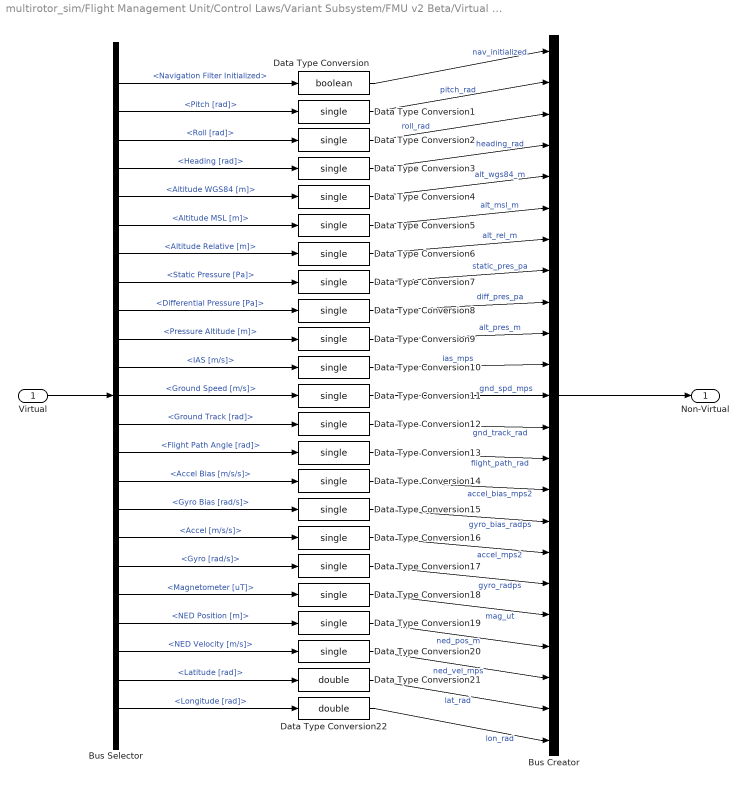
== system multirotor_sim/Flight Management Unit/Control Laws/Variant Subsystem/FMU v2 Beta/Virtual to Non-Virtual Mapping2 ==
  Virtual : Inport
  Bus Creator : BusCreator  Inputs=23  OutDataTypeStr=Bus: NavData  NonVirtualBus=on
  Bus Selector : BusSelector  OutputSignals=Navigation Filter Initialized,Pitch [rad],Roll [rad],Heading [rad],Altitude WGS84 [m],Altitude MSL [m],Altitude Relative [m],Static Pressure [Pa],Differential Pressure [Pa],Pressure Altitude [m],IAS [m/s],Ground Speed [m/s],Ground Track [rad],Flight Path Angle [rad],Accel Bias [m/s/s],Gyro Bias [rad/s],Accel [m/s/s],Gyro [rad/s],Magnetometer [uT],NED Position [m],NED Velocity [m/s],Latitude [rad],Longitude [rad]
  Data Type Conversion : DataTypeConversion  OutDataTypeStr=boolean
  Data Type Conversion{1..20} (20 alike) : DataTypeConversion  OutDataTypeStr=single
  Data Type Conversion21 : DataTypeConversion  OutDataTypeStr=double
  Data Type Conversion22 : DataTypeConversion  OutDataTypeStr=double
  Non-Virtual : Outport  OutDataTypeStr=Bus: NavData
  wires:
  Virtual/1 -> Bus Selector/1
  Bus Creator/1 -> Non-Virtual/1
  Bus Selector/1 -> Data Type Conversion/1  "<Navigation Filter Initialized>"
  Bus Selector/2 -> Data Type Conversion1/1  "<Pitch [rad]>"
  Bus Selector/3 -> Data Type Conversion2/1  "<Roll [rad]>"
  Bus Selector/4 -> Data Type Conversion3/1  "<Heading [rad]>"
  Bus Selector/5 -> Data Type Conversion4/1  "<Altitude WGS84 [m]>"
  Bus Selector/6 -> Data Type Conversion5/1  "<Altitude MSL [m]>"
  Bus Selector/7 -> Data Type Conversion6/1  "<Altitude Relative [m]>"
  Bus Selector/8 -> Data Type Conversion7/1  "<Static Pressure [Pa]>"
  Bus Selector/9 -> Data Type Conversion8/1  "<Differential Pressure [Pa]>"
  Bus Selector/10 -> Data Type Conversion9/1  "<Pressure Altitude [m]>"
  Bus Selector/11 -> Data Type Conversion10/1  "<IAS [m/s]>"
  Bus Selector/12 -> Data Type Conversion11/1  "<Ground Speed [m/s]>"
  Bus Selector/13 -> Data Type Conversion12/1  "<Ground Track [rad]>"
  Bus Selector/14 -> Data Type Conversion13/1  "<Flight Path Angle [rad]>"
  Bus Selector/15 -> Data Type Conversion14/1  "<Accel Bias [m/s/s]>"
  Bus Selector/16 -> Data Type Conversion15/1  "<Gyro Bias [rad/s]>"
  Bus Selector/17 -> Data Type Conversion16/1  "<Accel [m/s/s]>"
  Bus Selector/18 -> Data Type Conversion17/1  "<Gyro [rad/s]>"
  Bus Selector/19 -> Data Type Conversion18/1  "<Magnetometer [uT]>"
  Bus Selector/20 -> Data Type Conversion19/1  "<NED Position [m]>"
  Bus Selector/21 -> Data Type Conversion20/1  "<NED Velocity [m/s]>"
  Bus Selector/22 -> Data Type Conversion21/1  "<Latitude [rad]>"
  Bus Selector/23 -> Data Type Conversion22/1  "<Longitude [rad]>"
  Data Type Conversion/1 -> Bus Creator/1  "nav_initialized"
  Data Type Conversion1/1 -> Bus Creator/2  "pitch_rad"
  Data Type Conversion2/1 -> Bus Creator/3  "roll_rad"
  Data Type Conversion3/1 -> Bus Creator/4  "heading_rad"
  Data Type Conversion4/1 -> Bus Creator/5  "alt_wgs84_m"
  Data Type Conversion5/1 -> Bus Creator/6  "alt_msl_m"
  Data Type Conversion6/1 -> Bus Creator/7  "alt_rel_m"
  Data Type Conversion7/1 -> Bus Creator/8  "static_pres_pa"
  Data Type Conversion8/1 -> Bus Creator/9  "diff_pres_pa"
  Data Type Conversion9/1 -> Bus Creator/10  "alt_pres_m"
  Data Type Conversion10/1 -> Bus Creator/11  "ias_mps"
  Data Type Conversion11/1 -> Bus Creator/12  "gnd_spd_mps"
  Data Type Conversion12/1 -> Bus Creator/13  "gnd_track_rad"
  Data Type Conversion13/1 -> Bus Creator/14  "flight_path_rad"
  Data Type Conversion14/1 -> Bus Creator/15  "accel_bias_mps2"
  Data Type Conversion15/1 -> Bus Creator/16  "gyro_bias_radps"
  Data Type Conversion16/1 -> Bus Creator/17  "accel_mps2"
  Data Type Conversion18/1 -> Bus Creator/19  "mag_ut"
  Data Type Conversion19/1 -> Bus Creator/20  "ned_pos_m"
  Data Type Conversion20/1 -> Bus Creator/21  "ned_vel_mps"
  Data Type Conversion21/1 -> Bus Creator/22  "lat_rad"
  Data Type Conversion22/1 -> Bus Creator/23  "lon_rad"
  Data Type Conversion17/1 -> Bus Creator/18  "gyro_radps"

== system multirotor_sim/Flight Management Unit/Control Laws/Variant Subsystem/FMU v2 Beta/Virtual to Non-Virtual Mapping3 ==
  Virtual : Inport
  Bus Creator : BusCreator  Inputs=11  OutDataTypeStr=Bus: TelemData  NonVirtualBus=on
  Bus Selector : BusSelector  OutputSignals=Waypoints Updated,Fence Updated,Rally Points Updated,Current Waypoint Index,Number of Waypoints,Number of Fence Points,Number of Rally Points,Parameters,Flight Plan,Fence,Rally
  Data Type Conversion : DataTypeConversion  OutDataTypeStr=boolean
  Data Type Conversion1 : DataTypeConversion  OutDataTypeStr=boolean
  Data Type Conversion2 : DataTypeConversion  OutDataTypeStr=boolean
  Data Type Conversion{3..6} (4 alike) : DataTypeConversion  OutDataTypeStr=int16
  Data Type Conversion7 : DataTypeConversion  OutDataTypeStr=single
  Signal Conversion : SignalConversion  ConversionOutput=Nonvirtual bus  OverrideOpt=off
  Signal Conversion1 : SignalConversion  ConversionOutput=Nonvirtual bus  OverrideOpt=off
  Signal Conversion2 : SignalConversion  ConversionOutput=Nonvirtual bus  OverrideOpt=off
  Non-Virtual : Outport  OutDataTypeStr=Bus: TelemData
  wires:
  Virtual/1 -> Bus Selector/1
  Bus Creator/1 -> Non-Virtual/1
  Bus Selector/1 -> Data Type Conversion/1  "<Waypoints Updated>"
  Bus Selector/2 -> Data Type Conversion1/1  "<Fence Updated>"
  Bus Selector/3 -> Data Type Conversion2/1  "<Rally Points Updated>"
  Bus Selector/4 -> Data Type Conversion3/1  "<Current Waypoint Index>"
  Bus Selector/5 -> Data Type Conversion4/1  "<Number of Waypoints>"
  Bus Selector/6 -> Data Type Conversion5/1  "<Number of Fence Points>"
  Bus Selector/7 -> Data Type Conversion6/1  "<Number of Rally Points>"
  Bus Selector/8 -> Data Type Conversion7/1  "<Parameters>"
  Data Type Conversion/1 -> Bus Creator/1  "waypoints_updated"
  Data Type Conversion1/1 -> Bus Creator/2  "fence_updated"
  Data Type Conversion2/1 -> Bus Creator/3  "rally_points_updated"
  Data Type Conversion3/1 -> Bus Creator/4  "current_waypoint"
  Data Type Conversion4/1 -> Bus Creator/5  "num_waypoints"
  Data Type Conversion5/1 -> Bus Creator/6  "num_fence_items"
  Data Type Conversion6/1 -> Bus Creator/7  "num_rally_points"
  Data Type Conversion7/1 -> Bus Creator/8  "param"
  Bus Selector/9 -> Signal Conversion/1  "<Flight Plan>"
  Bus Selector/10 -> Signal Conversion1/1  "<Fence>"
  Bus Selector/11 -> Signal Conversion2/1  "<Rally>"
  Signal Conversion/1 -> Bus Creator/9  "flight_plan"
  Signal Conversion1/1 -> Bus Creator/10  "fence"
  Signal Conversion2/1 -> Bus Creator/11  "rally"

== system multirotor_sim/Flight Management Unit/Control Laws/Variant Subsystem/FMU v2 Beta/Virtual to Non-Virtual Mapping4 ==
  Non-Virtual : Inport  OutDataTypeStr=Bus: ControlData
  Bus Creator : BusCreator  Inputs=5
  Bus Selector : BusSelector  OutputSignals=waypoint_reached,mode,sbus,pwm,aux
  Data Type Conversion{1..4,22} (5 alike) : DataTypeConversion  OutDataTypeStr=double
  Virtual : Outport
  wires:
  Non-Virtual/1 -> Bus Selector/1
  Bus Creator/1 -> Virtual/1
  Bus Selector/1 -> Data Type Conversion22/1  "<waypoint_reached>"
  Data Type Conversion22/1 -> Bus Creator/1  "Waypoint Reached"
  Bus Selector/2 -> Data Type Conversion1/1  "<mode>"
  Data Type Conversion1/1 -> Bus Creator/2  "Mode"
  Bus Selector/3 -> Data Type Conversion2/1  "<sbus>"
  Data Type Conversion2/1 -> Bus Creator/3  "SBUS"
  Bus Selector/4 -> Data Type Conversion3/1  "<pwm>"
  Bus Selector/5 -> Data Type Conversion4/1  "<aux>"
  Data Type Conversion3/1 -> Bus Creator/4  "PWM"
  Data Type Conversion4/1 -> Bus Creator/5  "AUX"

== system multirotor_sim/Flight Management Unit/Sensor Models/GNSS/Triggered Subsystem/Norm ==
  2D Vector : Inport
  Product : Product
  Sqrt : Sqrt  SaturateOnIntegerOverflow=on
  Sum of Elements : Sum  Inputs=+
  Norm : Outport
  wires:
  2D Vector/1 -> Product/2, Product/1
  Product/1 -> Sum of Elements/1
  Sum of Elements/1 -> Sqrt/1
  Sqrt/1 -> Norm/1

== system multirotor_sim/Flight Management Unit/Control Laws/Variant Subsystem/FMU v1/Virtual to Non-Virtual Mapping1/Virtual to Non-Virtual Mapping1 ==
  Virtual : Inport
  Bus Creator : BusCreator  Inputs=10
  Bus Selector : BusSelector  OutputSignals=New Data,Lost Frame,Failsafe,Throttle Enable,Mode 0,Mode 1,Throttle,Pitch,Roll,Yaw
  Data Type Conversion{,1..3} (4 alike) : DataTypeConversion  OutDataTypeStr=boolean
  Data Type Conversion4 : DataTypeConversion  OutDataTypeStr=int8
  Data Type Conversion5 : DataTypeConversion  OutDataTypeStr=int8
  Data Type Conversion{6..9} (4 alike) : DataTypeConversion  OutDataTypeStr=single
  Non-Virtual : Outport  OutDataTypeStr=Bus: InceptorData
  wires:
  Data Type Conversion9/1 -> Bus Creator/10  "yaw"
  Data Type Conversion8/1 -> Bus Creator/9  "roll"
  Data Type Conversion7/1 -> Bus Creator/8  "pitch"
  Data Type Conversion6/1 -> Bus Creator/7  "throttle"
  Data Type Conversion5/1 -> Bus Creator/6  "mode1"
  Data Type Conversion4/1 -> Bus Creator/5  "mode0"
  Data Type Conversion3/1 -> Bus Creator/4  "throttle_en"
  Data Type Conversion2/1 -> Bus Creator/3  "failsafe"
  Data Type Conversion1/1 -> Bus Creator/2  "lost_frame"
  Bus Selector/10 -> Data Type Conversion9/1  "<Yaw>"
  Bus Selector/9 -> Data Type Conversion8/1  "<Roll>"
  Bus Selector/8 -> Data Type Conversion7/1  "<Pitch>"
  Bus Selector/7 -> Data Type Conversion6/1  "<Throttle>"
  Bus Selector/6 -> Data Type Conversion5/1  "<Mode 1>"
  Bus Selector/5 -> Data Type Conversion4/1  "<Mode 0>"
  Bus Selector/4 -> Data Type Conversion3/1  "<Throttle Enable>"
  Bus Selector/3 -> Data Type Conversion2/1  "<Failsafe>"
  Bus Selector/2 -> Data Type Conversion1/1  "<Lost Frame>"
  Data Type Conversion/1 -> Bus Creator/1  "new_data"
  Bus Selector/1 -> Data Type Conversion/1  "<New Data>"
  Bus Creator/1 -> Non-Virtual/1
  Virtual/1 -> Bus Selector/1

== system multirotor_sim/Flight Management Unit/Control Laws/Variant Subsystem/FMU v1/Virtual to Non-Virtual Mapping1/Virtual to Non-Virtual Mapping2 ==
  Virtual : Inport
  Bus Creator : BusCreator  Inputs=8
  Bus Selector : BusSelector  OutputSignals=New IMU Data,New Magnetometer Data,IMU Healthy,Magnetometer Healthy,Die Temperature [C],Accelerometer [m/s/s],Gyro [rad/s],Magnetometer [uT]
  Data Type Conversion{,1..3} (4 alike) : DataTypeConversion  OutDataTypeStr=boolean
  Data Type Conversion{4..7} (4 alike) : DataTypeConversion  OutDataTypeStr=single
  Non-Virtual : Outport  OutDataTypeStr=Bus: ImuData
  wires:
  Data Type Conversion7/1 -> Bus Creator/8  "mag_ut"
  Data Type Conversion6/1 -> Bus Creator/7  "gyro_radps"
  Data Type Conversion5/1 -> Bus Creator/6  "accel_mps2"
  Bus Selector/8 -> Data Type Conversion7/1  "<Magnetometer [uT]>"
  Bus Selector/7 -> Data Type Conversion6/1  "<Gyro [rad/s]>"
  Bus Selector/6 -> Data Type Conversion5/1  "<Accelerometer [m/s/s]>"
  Data Type Conversion4/1 -> Bus Creator/5  "die_temp_c"
  Bus Selector/5 -> Data Type Conversion4/1  "<Die Temperature [C]>"
  Data Type Conversion3/1 -> Bus Creator/4  "mag_healthy"
  Bus Selector/4 -> Data Type Conversion3/1  "<Magnetometer Healthy>"
  Data Type Conversion2/1 -> Bus Creator/3  "imu_healthy"
  Bus Selector/3 -> Data Type Conversion2/1  "<IMU Healthy>"
  Data Type Conversion1/1 -> Bus Creator/2  "new_mag_data"
  Bus Selector/2 -> Data Type Conversion1/1  "<New Magnetometer Data>"
  Data Type Conversion/1 -> Bus Creator/1  "new_imu_data"
  Bus Selector/1 -> Data Type Conversion/1  "<New IMU Data>"
  Virtual/1 -> Bus Selector/1
  Bus Creator/1 -> Non-Virtual/1
